simulink model "ZEPS"  (R2021b)
settings: Solver=VariableStepAuto  StartTime=0.0  StopTime=432000  FixedStep=1/60/60  RelTol=1e-3
model workspace: external: MATLAB File modelWorkspace.m (data not in the file)
values from neighbouring files (symbols this model uses):
  controlBT = 1    [modelWorkspace.m]
  controlEng = 1    [modelWorkspace.m]
  controlFC = 0    [modelWorkspace.m]
  controlFW = 0    [modelWorkspace.m]
  controlHS = 1    [modelWorkspace.m]
  controlSol = 0    [modelWorkspace.m]
  controlW = 0    [modelWorkspace.m]
  controlWW = 0    [modelWorkspace.m]
  data = get_scenario(scenario)    [UpdateModel.m]    (also in f_import_PEL.m = rmmissing(data,1,'MinNumMissing',10); get_scenario.m = data(timerange(datetime(FROM, 'InputFormat', 'dd.MM.yyyy HH:; thesis_images.m = get_scenario(1))
  sun = sun(sun.Date>date,:)    [get_irradiance.m]    (also in get_solar_from_file.m = sun(timerange(FROM+dt, TO+dt),:); thesis_images.m = get_irradiance(50, 14, "01.01.2016"))
undefined symbols (not defined in the file or in its folder): days, Ion, Lithium, seconds
libraries: mylib x15, simulink x5, spsControlledCurrentSourceLib x5, spsVoltageMeasurementLib x5, spsBatteryLib x1, simulink_extras x1, spspowerguiLib x1
settings Model: PacingRate=3600  VariantFading=off  Creator=janluca  LastModifiedBy=janluca
settings SolverCC: ZeroCrossAlgorithm=Adaptive  AlgebraicLoopSolver=LineSearch
settings DebuggingCC: AlgebraicLoopMsg=none  IgnoredZcDiagnostic=none  SFMachineParentedDataDiag=warning

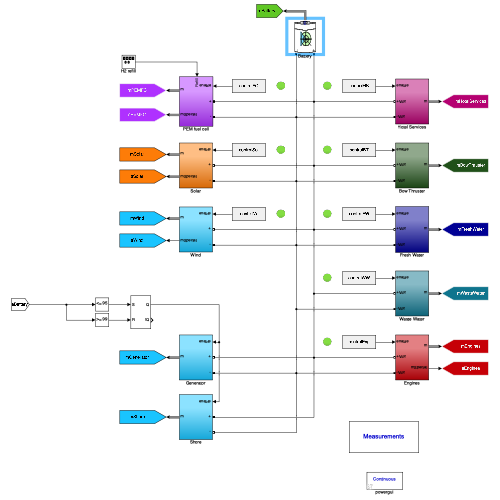
[thumbnail: Simulink's stored preview of the top-level diagram]
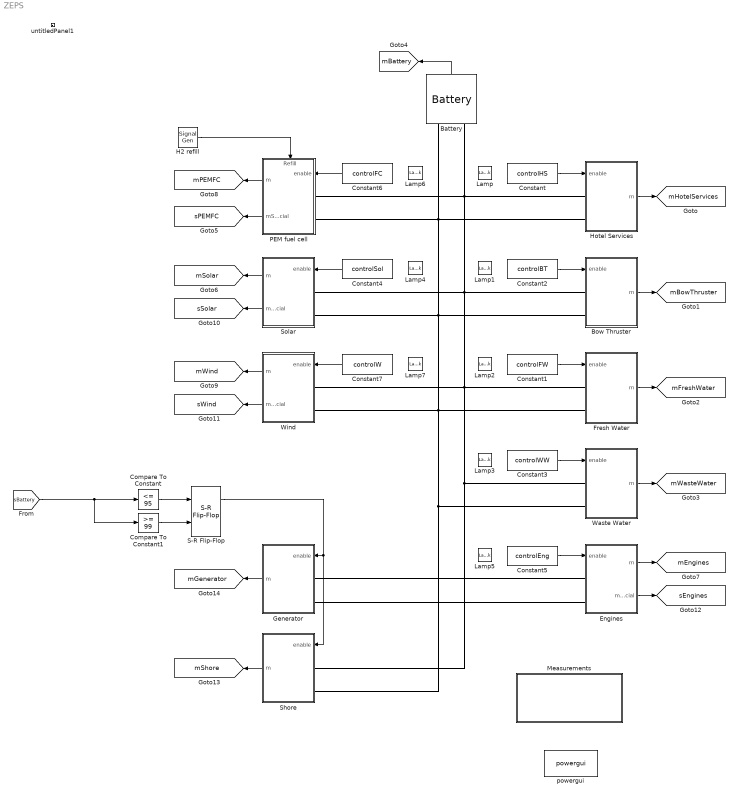
== system ZEPS ==
  Battery : spsBatteryLib/Battery  BatType=Lithium-Ion  ShowTempParam=off  ThermalPreset=no  ShowAgeParam=off  NomV=38.4*21  NomQ=100*50  SOC=90  Batt_Tr=0.1  PresetModel=off  MaxQ=125*50  MinV=30*21  FullV=42*21  Dis_rate=50*50  R=0.0024828  Normal_OP=100*50  expZone=[837.9 2500]  current=[20 100 200]  Units=Time  Tci=20  NomT=20  T2=-30  MaxQ2=4.8  FullV2=7.1  Normal_OP2=5.655  expZone2="[6.58           1]"  Rca=0.6  ti=2000  Dp=0  Neq0=0  Tsim=1e6  Ta1=25  Qeol=5.4*0.9  Reol=0.013333*1.2  Char_age=[2.3478, 3]  Dis_age=[2.3478, 10]  N1=1500  N2=10500  N3=1000  N4=1400  Ta2=45  N5=950
  Bow Thruster : Subsystem
  Compare To Constant : simulink/Logic and Bit Operations/Compare To Constant  relop=<=  const=95  OutDataTypeStr=boolean
  Compare To Constant1 : simulink/Logic and Bit Operations/Compare To Constant  relop=>=  const=99  OutDataTypeStr=boolean
  Constant : Constant  Value=controlHS
  Constant1 : Constant  Value=controlFW
  Constant2 : Constant  Value=controlBT
  Constant3 : Constant  Value=controlWW
  Constant4 : Constant  Value=controlSol
  Constant5 : Constant  Value=controlEng
  Constant6 : Constant  Value=controlFC
  Constant7 : Constant  Value=controlW
  Engines : Subsystem
  Fresh Water : Subsystem
  Generator : Subsystem
      settings: PortSchema="{\"entries\":[{\"content\":{\"sides\":[{\"content\":{\"connectorIds\":[\"Out1\"]},\"type\":\"ConnectorPlacement.EquallySpacedRectSide\",\"uuid\":\"11c6df83-a77d-42e1-93c3-7e92626e8295\"},{\"content\":{\"connectorIds\":[\"In1\",\"RConn1\",\"RConn2\"],\"side\":\"RIGHT\"},\"type\":\"ConnectorPlacement.EquallySpacedRectSide\",\"uuid\":\"be484aa3-b470-4b9a-a56f-17a6492ffa37\"},{\"content\":{\"connectorIds\":[],\"side\":\"TOP\"},\"type\":\"ConnectorPlacement.EquallySpacedRectSide\",\"uuid\":\"b9721f03-f883-4f0f-ae4c-83e5c2ad9b8b\"},{\"content\":{\"connectorIds\":[],\"side\":\"HIDDEN\"},\"type\":\"ConnectorPlacement.EquallySpacedRectSide\",\"uuid\":\"b91deee7-9db2-4cb3-a16e-378b8e6a58a6\"}]},\"type\":\"ConnectorPlacement.EquallySpacedConnector\",\"uuid\":\"590b808f-ca80-4a0b-b9c9-4d18c7197559\"}],\"packageUris\":[\"http://schema.mathworks.com/mf0/Connector/R2020b\"],\"version\":\"1.0\"}"
  H2 refill : SignalGenerator  WaveForm=sawtooth  Amplitude=0  Frequency=1/seconds(days(1))
  Hotel Services : Subsystem
  Lamp{,1..7} (8 alike) : LampBlock  LabelPosition=Hide
  Measurements : Subsystem
      mask Display: color('blue');disp('Measurements')
  PEM fuel cell : Subsystem
      settings: PortSchema="{\"entries\":[{\"content\":{\"sides\":[{\"content\":{\"connectorIds\":[\"Out1\",\"Out2\"]},\"type\":\"ConnectorPlacement.EquallySpacedRectSide\",\"uuid\":\"11c6df83-a77d-42e1-93c3-7e92626e8295\"},{\"content\":{\"connectorIds\":[\"In2\",\"RConn1\",\"RConn2\"],\"side\":\"RIGHT\"},\"type\":\"ConnectorPlacement.EquallySpacedRectSide\",\"uuid\":\"be484aa3-b470-4b9a-a56f-17a6492ffa37\"},{\"content\":{\"connectorIds\":[\"In1\"],\"side\":\"TOP\"},\"type\":\"ConnectorPlacement.EquallySpacedRectSide\",\"uuid\":\"b9721f03-f883-4f0f-ae4c-83e5c2ad9b8b\"},{\"content\":{\"connectorIds\":[],\"side\":\"HIDDEN\"},\"type\":\"ConnectorPlacement.EquallySpacedRectSide\",\"uuid\":\"b91deee7-9db2-4cb3-a16e-378b8e6a58a6\"}]},\"type\":\"ConnectorPlacement.EquallySpacedConnector\",\"uuid\":\"590b808f-ca80-4a0b-b9c9-4d18c7197559\"}],\"packageUris\":[\"http://schema.mathworks.com/mf0/Connector/R2020b\"],\"version\":\"1.0\"}"
  S-R Flip-Flop : simulink_extras/Flip Flops/S-R Flip-Flop  initial_condition=0
  Shore : Subsystem
      settings: PortSchema="{\"entries\":[{\"content\":{\"sides\":[{\"content\":{\"connectorIds\":[\"Out1\"]},\"type\":\"ConnectorPlacement.EquallySpacedRectSide\",\"uuid\":\"11c6df83-a77d-42e1-93c3-7e92626e8295\"},{\"content\":{\"connectorIds\":[\"In1\",\"RConn1\",\"RConn2\"],\"side\":\"RIGHT\"},\"type\":\"ConnectorPlacement.EquallySpacedRectSide\",\"uuid\":\"be484aa3-b470-4b9a-a56f-17a6492ffa37\"},{\"content\":{\"connectorIds\":[],\"side\":\"TOP\"},\"type\":\"ConnectorPlacement.EquallySpacedRectSide\",\"uuid\":\"b9721f03-f883-4f0f-ae4c-83e5c2ad9b8b\"},{\"content\":{\"connectorIds\":[],\"side\":\"HIDDEN\"},\"type\":\"ConnectorPlacement.EquallySpacedRectSide\",\"uuid\":\"b91deee7-9db2-4cb3-a16e-378b8e6a58a6\"}]},\"type\":\"ConnectorPlacement.EquallySpacedConnector\",\"uuid\":\"590b808f-ca80-4a0b-b9c9-4d18c7197559\"}],\"packageUris\":[\"http://schema.mathworks.com/mf0/Connector/R2020b\"],\"version\":\"1.0\"}"
  Solar : Subsystem
      settings: PortSchema="{\"entries\":[{\"content\":{\"sides\":[{\"content\":{\"connectorIds\":[\"Out1\",\"Out2\"]},\"type\":\"ConnectorPlacement.EquallySpacedRectSide\",\"uuid\":\"11c6df83-a77d-42e1-93c3-7e92626e8295\"},{\"content\":{\"connectorIds\":[\"In1\",\"RConn1\",\"RConn2\"],\"side\":\"RIGHT\"},\"type\":\"ConnectorPlacement.EquallySpacedRectSide\",\"uuid\":\"be484aa3-b470-4b9a-a56f-17a6492ffa37\"},{\"content\":{\"connectorIds\":[],\"side\":\"TOP\"},\"type\":\"ConnectorPlacement.EquallySpacedRectSide\",\"uuid\":\"b9721f03-f883-4f0f-ae4c-83e5c2ad9b8b\"},{\"content\":{\"connectorIds\":[],\"side\":\"HIDDEN\"},\"type\":\"ConnectorPlacement.EquallySpacedRectSide\",\"uuid\":\"b91deee7-9db2-4cb3-a16e-378b8e6a58a6\"}]},\"type\":\"ConnectorPlacement.EquallySpacedConnector\",\"uuid\":\"590b808f-ca80-4a0b-b9c9-4d18c7197559\"}],\"packageUris\":[\"http://schema.mathworks.com/mf0/Connector/R2020b\"],\"version\":\"1.0\"}"
  Waste Water : Subsystem
  Wind : Subsystem
      settings: PortSchema="{\"entries\":[{\"content\":{\"sides\":[{\"content\":{\"connectorIds\":[\"Out1\",\"Out2\"]},\"type\":\"ConnectorPlacement.EquallySpacedRectSide\",\"uuid\":\"11c6df83-a77d-42e1-93c3-7e92626e8295\"},{\"content\":{\"connectorIds\":[\"In1\",\"RConn1\",\"RConn2\"],\"side\":\"RIGHT\"},\"type\":\"ConnectorPlacement.EquallySpacedRectSide\",\"uuid\":\"be484aa3-b470-4b9a-a56f-17a6492ffa37\"},{\"content\":{\"connectorIds\":[],\"side\":\"TOP\"},\"type\":\"ConnectorPlacement.EquallySpacedRectSide\",\"uuid\":\"b9721f03-f883-4f0f-ae4c-83e5c2ad9b8b\"},{\"content\":{\"connectorIds\":[],\"side\":\"HIDDEN\"},\"type\":\"ConnectorPlacement.EquallySpacedRectSide\",\"uuid\":\"b91deee7-9db2-4cb3-a16e-378b8e6a58a6\"}]},\"type\":\"ConnectorPlacement.EquallySpacedConnector\",\"uuid\":\"590b808f-ca80-4a0b-b9c9-4d18c7197559\"}],\"packageUris\":[\"http://schema.mathworks.com/mf0/Connector/R2020b\"],\"version\":\"1.0\"}"
  powergui : spspowerguiLib/powergui  Priority=1  SimulationMode=Continuous  SampleTime=60  frequency=60  Iterations=50  frequencyindice=0  Pbase=100e6  ErrMax=1e-4  UnitsV=kV  UnitsW=MW  buscounter=0  FunctionMessages=off  echomessages=off  EnableUseOfTLC=off  CurrentSourceSwitches=off  DisableSnubberDevices=off  DisableRonSwitches=off  DisableVfSwitches=off  DisplayEquations=off  AutomaticDiscreteSolvers=off  SolverType=Tustin/Backward Euler (TBE)  Interpol=off  ExternalGateDelay=off  methode=off  Ts=100  x0status=blocks  SPID=on  SwTol=0  HookPort=off  NonlinearTolerance=1e-4  nMaxIteration=100  ContinueOnMaxIteration=off  RestoreLinks=warning  ResistiveCurrentMeasurement=off  Frange=[0:2:500]  Ylog=off  Xlog=on  ShowGrid=off  save=off  variable=ZData  structure=0  ZoomFFT=off  StartTime=0.0  cycles=1  DisplayStyle=1  fundamental=60  FreqAxis=off  MaxFrequency=1000  frequencyindicesteady=1  RmsSteady=1  display=off
  untitledPanel1 : Subsystem  Tag=HiddenForWebPanel  IsWebBlockPanel=on
  tag scope: mBattery=global, mBowThruster=global, mEngines=global, mFreshWater=global, mGenerator=global, mHotelServices=global, mPEMFC=global, mShore=global, mSolar=global, mWasteWater=global, mWind=global, sEngines=global, sPEMFC=global, sSolar=global, sWind=global
  wires:
  Constant/1 -> Hotel Services/1(enable)
  Hotel Services/1(m) -> [mHotelServices]
  Bow Thruster/1(m) -> [mBowThruster]
  Fresh Water/1(m) -> [mFreshWater]
  Waste Water/1(m) -> [mWasteWater]
  Battery/1 -> [mBattery]
  Constant2/1 -> Bow Thruster/1(enable)
  Constant1/1 -> Fresh Water/1(enable)
  Constant3/1 -> Waste Water/1(enable)
  Solar/1(m) -> [mSolar]
  Constant4/1 -> Solar/1(enable)
  Constant5/1 -> Engines/1(enable)
  Engines/1(m) -> [mEngines]
  PEM fuel cell/1(m) -> [mPEMFC]
  Constant6/1 -> PEM fuel cell/2(enable)
  Wind/1(m) -> [mWind]
  Constant7/1 -> Wind/1(enable)
  PEM fuel cell/2(mSpecial) -> [sPEMFC]
  Solar/2(mSpecial) -> [sSolar]
  Wind/2(mSpecial) -> [sWind]
  Engines/2(mSpecial) -> [sEngines]
  H2 refill/1 -> PEM fuel cell/1(Refill)
  Generator/1(m) -> [mGenerator]
  Compare To Constant/1 -> S-R Flip-Flop/1
  [sBattery] -> Compare To Constant1/1, Compare To Constant/1
  Compare To Constant1/1 -> S-R Flip-Flop/2
  S-R Flip-Flop/1 -> Shore/1(enable), Generator/1(enable)
  Shore/1(m) -> [mShore]
  connections:
  Hotel Services/LConn1 -- Shore/RConn1 -- Engines/LConn1 -- Generator/RConn1 -- Waste Water/LConn1 -- Wind/RConn1 -- Fresh Water/LConn1 -- Solar/RConn1 -- Bow Thruster/LConn1 -- PEM fuel cell/RConn1 -- Battery/LConn1
  Hotel Services/LConn2 -- Wind/RConn2 -- Shore/RConn2 -- Engines/LConn2 -- Generator/RConn2 -- Waste Water/LConn2 -- Fresh Water/LConn2 -- Solar/RConn2 -- Bow Thruster/LConn2 -- PEM fuel cell/RConn2 -- Battery/LConn2

== system ZEPS/Bow Thruster ==
  enable : Inport
  AC converter simple : mylib/AC converter simple  eff=0.98
  Clock : Clock
  Constant : Constant  Value=0
  Load Data power bow thruster : Lookup_n-D  NumberOfTableDimensions=1  BreakpointsForDimension1=data.time  BeginIndexSearchUsingPreviousIndexResult=on  Table=data.P_BT  InternalRulePriority=Speed  RndMeth=Simplest  InputSameDT=on
  Switch : Switch  Criteria=u2 > Threshold
  VI measurement : mylib/VI measurement  SystemSampleTime=-1  VariantActivationTime=update diagram  Latency=0  AutoFrameSizeCalculation=off
      settings: PortSchema="{\"entries\":[{\"content\":{\"sides\":[{\"content\":{\"connectorIds\":[\"LConn1\",\"LConn2\"]},\"type\":\"ConnectorPlacement.EquallySpacedRectSide\",\"uuid\":\"f3b73344-d0cf-4b93-ad96-f780fa5a1256\"},{\"content\":{\"connectorIds\":[\"RConn1\",\"RConn2\"],\"side\":\"RIGHT\"},\"type\":\"ConnectorPlacement.EquallySpacedRectSide\",\"uuid\":\"030ebb8c-daa3-4185-a78c-b002204e2a62\"},{\"content\":{\"connectorIds\":[\"Out1\"],\"side\":\"TOP\"},\"type\":\"ConnectorPlacement.EquallySpacedRectSide\",\"uuid\":\"0cc05069-4c24-40a7-976e-8b87ed915541\"},{\"content\":{\"connectorIds\":[],\"side\":\"HIDDEN\"},\"type\":\"ConnectorPlacement.EquallySpacedRectSide\",\"uuid\":\"da030f82-010e-483f-97d7-c36c3edfce40\"}]},\"type\":\"ConnectorPlacement.EquallySpacedConnector\",\"uuid\":\"1bb0f634-fa5d-4f47-8259-a0e02a201bbc\"}],\"packageUris\":[\"http://schema.mathworks.com/mf0/Connector/R2020b\"],\"version\":\"1.0\"}"
  +Vdc : PMIOPort  Tag=PMCPort  Side=Left
  -Vdc : PMIOPort  Tag=PMCPort  Port=2  Side=Left
  m : Outport
  wires:
  Switch/1 -> AC converter simple/1
  VI measurement/1 -> m/1
  Clock/1 -> Load Data power bow thruster/1
  enable/1 -> Switch/2
  Constant/1 -> Switch/3
  Load Data power bow thruster/1 -> Switch/1
  connections:
  VI measurement/LConn1 -- AC converter simple/RConn1
  +Vdc/RConn1 -- VI measurement/RConn1
  -Vdc/RConn1 -- VI measurement/RConn2
  VI measurement/LConn2 -- AC converter simple/RConn2

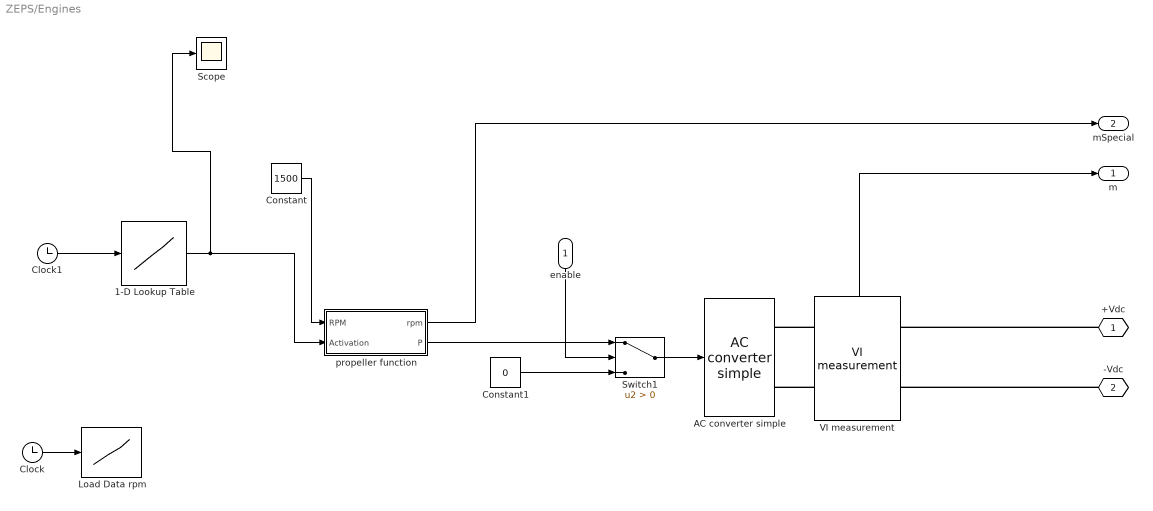
== system ZEPS/Engines ==
  enable : Inport
  1-D Lookup Table : Lookup_n-D  NumberOfTableDimensions=1  BreakpointsForDimension1="3600* [0   2    21    24    43    49    68    72    91    97   116   119   138   143]"  Table="600*[1    0    1     0     1     0     1     0     1     0     1     0     1     0]"  InterpMethod=Flat  InternalRulePriority=Speed  RndMeth=Simplest  InputSameDT=on
  AC converter simple : mylib/AC converter simple  eff=0.98
  Clock : Clock
  Clock1 : Clock
  Constant : Constant  Value=1500
  Constant1 : Constant  Value=0
  Load Data rpm : Lookup_n-D  NumberOfTableDimensions=1  BreakpointsForDimension1=data.time  BeginIndexSearchUsingPreviousIndexResult=on  Table=data.rpm  InternalRulePriority=Speed  RndMeth=Simplest  InputSameDT=on
  Scope : Scope
  Switch1 : Switch  Criteria=u2 > Threshold
  VI measurement : mylib/VI measurement  SystemSampleTime=-1  VariantActivationTime=update diagram  Latency=0  AutoFrameSizeCalculation=off
      settings: PortSchema="{\"entries\":[{\"content\":{\"sides\":[{\"content\":{\"connectorIds\":[\"LConn1\",\"LConn2\"]},\"type\":\"ConnectorPlacement.EquallySpacedRectSide\",\"uuid\":\"f3b73344-d0cf-4b93-ad96-f780fa5a1256\"},{\"content\":{\"connectorIds\":[\"RConn1\",\"RConn2\"],\"side\":\"RIGHT\"},\"type\":\"ConnectorPlacement.EquallySpacedRectSide\",\"uuid\":\"030ebb8c-daa3-4185-a78c-b002204e2a62\"},{\"content\":{\"connectorIds\":[\"Out1\"],\"side\":\"TOP\"},\"type\":\"ConnectorPlacement.EquallySpacedRectSide\",\"uuid\":\"0cc05069-4c24-40a7-976e-8b87ed915541\"},{\"content\":{\"connectorIds\":[],\"side\":\"HIDDEN\"},\"type\":\"ConnectorPlacement.EquallySpacedRectSide\",\"uuid\":\"da030f82-010e-483f-97d7-c36c3edfce40\"}]},\"type\":\"ConnectorPlacement.EquallySpacedConnector\",\"uuid\":\"1bb0f634-fa5d-4f47-8259-a0e02a201bbc\"}],\"packageUris\":[\"http://schema.mathworks.com/mf0/Connector/R2020b\"],\"version\":\"1.0\"}"
  propeller function : Subsystem
  +Vdc : PMIOPort  Tag=PMCPort  Side=Left
  -Vdc : PMIOPort  Tag=PMCPort  Port=2  Side=Left
  m : Outport
  mSpecial : Outport  Port=2
  wires:
  Clock/1 -> Load Data rpm/1
  Switch1/1 -> AC converter simple/1
  Constant1/1 -> Switch1/3
  propeller function/2(P) -> Switch1/1
  enable/1 -> Switch1/2
  VI measurement/1 -> m/1
  propeller function/1(rpm) -> mSpecial/1
  Clock1/1 -> 1-D Lookup Table/1
  Constant/1 -> propeller function/1(RPM)
  1-D Lookup Table/1 -> propeller function/2(Activation), Scope/1
  connections:
  VI measurement/LConn1 -- AC converter simple/RConn1
  -Vdc/RConn1 -- VI measurement/RConn2
  VI measurement/LConn2 -- AC converter simple/RConn2
  +Vdc/RConn1 -- VI measurement/RConn1

== system ZEPS/Fresh Water ==
  enable : Inport
  AC converter simple : mylib/AC converter simple  eff=0.98
  Constant : Constant  Value=0
  Power : Constant  Value=2300
  Switch : Switch  Criteria=u2 > Threshold
  VI measurement : mylib/VI measurement  SystemSampleTime=-1  VariantActivationTime=update diagram  Latency=0  AutoFrameSizeCalculation=off
      settings: PortSchema="{\"entries\":[{\"content\":{\"sides\":[{\"content\":{\"connectorIds\":[\"LConn1\",\"LConn2\"]},\"type\":\"ConnectorPlacement.EquallySpacedRectSide\",\"uuid\":\"f3b73344-d0cf-4b93-ad96-f780fa5a1256\"},{\"content\":{\"connectorIds\":[\"RConn1\",\"RConn2\"],\"side\":\"RIGHT\"},\"type\":\"ConnectorPlacement.EquallySpacedRectSide\",\"uuid\":\"030ebb8c-daa3-4185-a78c-b002204e2a62\"},{\"content\":{\"connectorIds\":[\"Out1\"],\"side\":\"TOP\"},\"type\":\"ConnectorPlacement.EquallySpacedRectSide\",\"uuid\":\"0cc05069-4c24-40a7-976e-8b87ed915541\"},{\"content\":{\"connectorIds\":[],\"side\":\"HIDDEN\"},\"type\":\"ConnectorPlacement.EquallySpacedRectSide\",\"uuid\":\"da030f82-010e-483f-97d7-c36c3edfce40\"}]},\"type\":\"ConnectorPlacement.EquallySpacedConnector\",\"uuid\":\"1bb0f634-fa5d-4f47-8259-a0e02a201bbc\"}],\"packageUris\":[\"http://schema.mathworks.com/mf0/Connector/R2020b\"],\"version\":\"1.0\"}"
  +Vdc : PMIOPort  Tag=PMCPort  Side=Left
  -Vdc : PMIOPort  Tag=PMCPort  Port=2  Side=Left
  m : Outport
  wires:
  VI measurement/1 -> m/1
  enable/1 -> Switch/2
  Constant/1 -> Switch/3
  Power/1 -> Switch/1
  Switch/1 -> AC converter simple/1
  connections:
  VI measurement/LConn1 -- AC converter simple/RConn1
  VI measurement/LConn2 -- AC converter simple/RConn2
  +Vdc/RConn1 -- VI measurement/RConn1
  -Vdc/RConn1 -- VI measurement/RConn2

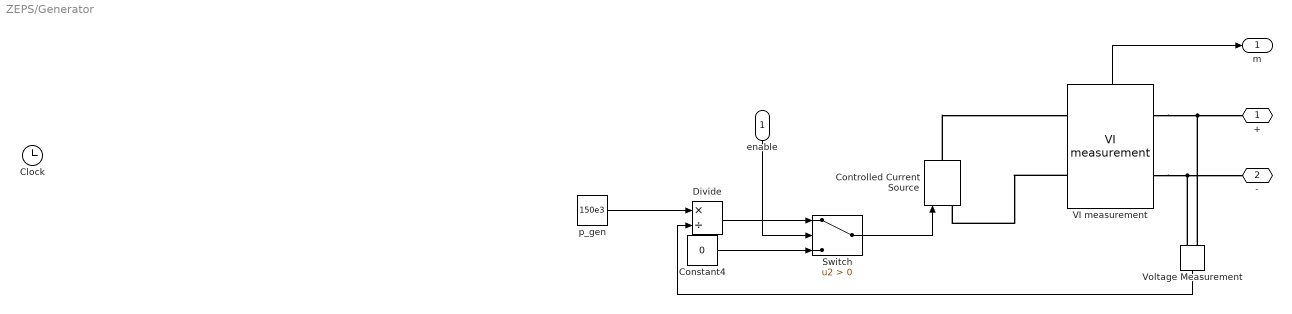
== system ZEPS/Generator ==
  enable : Inport
  Clock : Clock
  Constant4 : Constant  Value=0
  Controlled Current Source : spsControlledCurrentSourceLib/Controlled Current Source  Initialize=on  Source_Type=AC  Amplitude=0  Phase=0  Frequency=0  Measurements=None
  Divide : Product  Inputs=*/
  Switch : Switch  Criteria=u2 > Threshold
  VI measurement : mylib/VI measurement  SystemSampleTime=-1  VariantActivationTime=update diagram  Latency=0  AutoFrameSizeCalculation=off
      settings: PortSchema="{\"entries\":[{\"content\":{\"sides\":[{\"content\":{\"connectorIds\":[\"LConn1\",\"LConn2\"]},\"type\":\"ConnectorPlacement.EquallySpacedRectSide\",\"uuid\":\"f3b73344-d0cf-4b93-ad96-f780fa5a1256\"},{\"content\":{\"connectorIds\":[\"RConn1\",\"RConn2\"],\"side\":\"RIGHT\"},\"type\":\"ConnectorPlacement.EquallySpacedRectSide\",\"uuid\":\"030ebb8c-daa3-4185-a78c-b002204e2a62\"},{\"content\":{\"connectorIds\":[\"Out1\"],\"side\":\"TOP\"},\"type\":\"ConnectorPlacement.EquallySpacedRectSide\",\"uuid\":\"0cc05069-4c24-40a7-976e-8b87ed915541\"},{\"content\":{\"connectorIds\":[],\"side\":\"HIDDEN\"},\"type\":\"ConnectorPlacement.EquallySpacedRectSide\",\"uuid\":\"da030f82-010e-483f-97d7-c36c3edfce40\"}]},\"type\":\"ConnectorPlacement.EquallySpacedConnector\",\"uuid\":\"1bb0f634-fa5d-4f47-8259-a0e02a201bbc\"}],\"packageUris\":[\"http://schema.mathworks.com/mf0/Connector/R2020b\"],\"version\":\"1.0\"}"
  Voltage Measurement : spsVoltageMeasurementLib/Voltage Measurement  PhasorSimulation=off  OutputType=Complex  PSBequivalent=0
  p_gen : Constant  Value=150e3
  + : PMIOPort  Side=Right
  - : PMIOPort  Port=2  Side=Right
  m : Outport
  wires:
  Switch/1 -> Controlled Current Source/1
  enable/1 -> Switch/2
  Constant4/1 -> Switch/3
  Divide/1 -> Switch/1
  VI measurement/1 -> m/1
  Voltage Measurement/1 -> Divide/2
  p_gen/1 -> Divide/1
  connections:
  VI measurement/LConn1 -- Voltage Measurement/LConn1 -- +/RConn1
  VI measurement/LConn2 -- Voltage Measurement/LConn2 -- -/RConn1
  VI measurement/RConn2 -- Controlled Current Source/LConn1
  Controlled Current Source/RConn1 -- VI measurement/RConn1

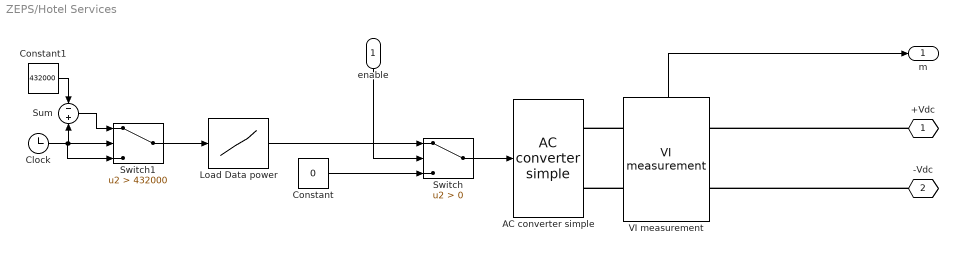
== system ZEPS/Hotel Services ==
  enable : Inport
  AC converter simple : mylib/AC converter simple  eff=0.98
  Clock : Clock
  Constant : Constant  Value=0
  Constant1 : Constant  Value=432000
  Load Data power : Lookup_n-D  NumberOfTableDimensions=1  BreakpointsForDimension1=data.time  BeginIndexSearchUsingPreviousIndexResult=on  Table=data.P  InternalRulePriority=Speed  RndMeth=Simplest  InputSameDT=on
  Sum : Sum  Inputs=-|+
  Switch : Switch  Criteria=u2 > Threshold
  Switch1 : Switch  Criteria=u2 > Threshold  Threshold=432000
  VI measurement : mylib/VI measurement  SystemSampleTime=-1  VariantActivationTime=update diagram  Latency=0  AutoFrameSizeCalculation=off
      settings: PortSchema="{\"entries\":[{\"content\":{\"sides\":[{\"content\":{\"connectorIds\":[\"LConn1\",\"LConn2\"]},\"type\":\"ConnectorPlacement.EquallySpacedRectSide\",\"uuid\":\"f3b73344-d0cf-4b93-ad96-f780fa5a1256\"},{\"content\":{\"connectorIds\":[\"RConn1\",\"RConn2\"],\"side\":\"RIGHT\"},\"type\":\"ConnectorPlacement.EquallySpacedRectSide\",\"uuid\":\"030ebb8c-daa3-4185-a78c-b002204e2a62\"},{\"content\":{\"connectorIds\":[\"Out1\"],\"side\":\"TOP\"},\"type\":\"ConnectorPlacement.EquallySpacedRectSide\",\"uuid\":\"0cc05069-4c24-40a7-976e-8b87ed915541\"},{\"content\":{\"connectorIds\":[],\"side\":\"HIDDEN\"},\"type\":\"ConnectorPlacement.EquallySpacedRectSide\",\"uuid\":\"da030f82-010e-483f-97d7-c36c3edfce40\"}]},\"type\":\"ConnectorPlacement.EquallySpacedConnector\",\"uuid\":\"1bb0f634-fa5d-4f47-8259-a0e02a201bbc\"}],\"packageUris\":[\"http://schema.mathworks.com/mf0/Connector/R2020b\"],\"version\":\"1.0\"}"
  +Vdc : PMIOPort  Tag=PMCPort  Side=Left
  -Vdc : PMIOPort  Tag=PMCPort  Port=2  Side=Left
  m : Outport
  wires:
  Load Data power/1 -> Switch/1
  enable/1 -> Switch/2
  Switch/1 -> AC converter simple/1
  VI measurement/1 -> m/1
  Constant/1 -> Switch/3
  Clock/1 -> Sum/2, Switch1/2, Switch1/3
  Switch1/1 -> Load Data power/1
  Sum/1 -> Switch1/1
  Constant1/1 -> Sum/1
  connections:
  VI measurement/LConn1 -- AC converter simple/RConn1
  VI measurement/LConn2 -- AC converter simple/RConn2
  +Vdc/RConn1 -- VI measurement/RConn1
  -Vdc/RConn1 -- VI measurement/RConn2

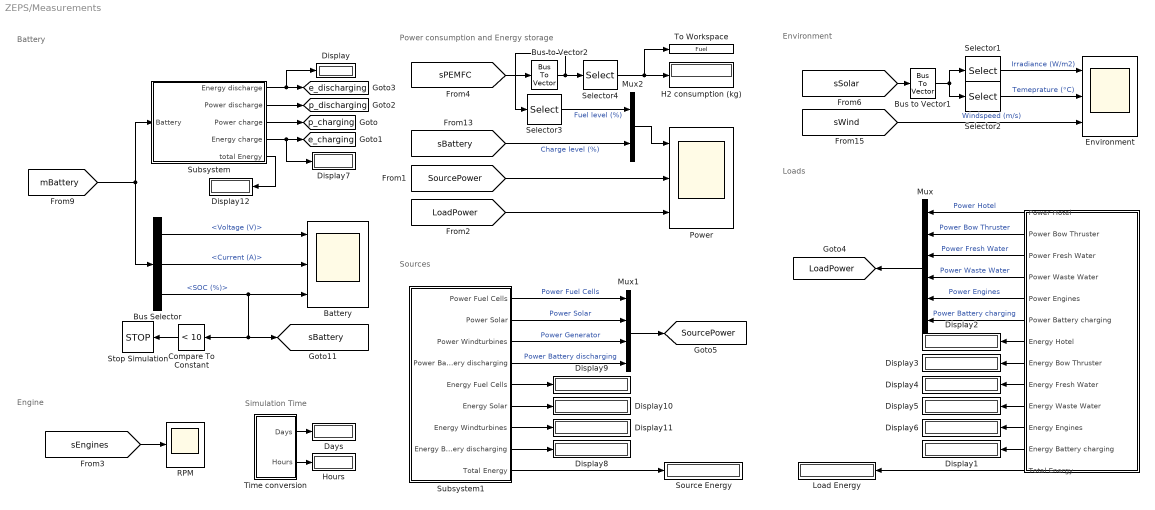
== system ZEPS/Measurements ==
  note: Engine
  note: Environment
  note: Power consumption and Energy storage
  note: Sources
  note: Loads
  note: Simulation Time
  note: Battery
  " " : Subsystem
  Battery : Scope  NumInputPorts=3
  Bus Selector : BusSelector  OutputSignals=Voltage (V),Current (A),SOC (%)
  Bus to Vector1 : BusToVector
  Bus to Vector2 : BusToVector
  Compare To Constant : simulink/Logic and Bit Operations/Compare To Constant  relop=<  const=10  OutDataTypeStr=boolean
  Days : Display
      settings: Format=bank
  Display{,1..12} (13 alike) : Display
  Environment : Scope  NumInputPorts=3
  H2 consumption (kg) : Display
  Hours : Display
      settings: Format=bank
  Load Energy : Display
      settings: Format=bank
  Mux : Mux  Inputs=6
  Mux1 : Mux
  Mux2 : Mux  Inputs=2
  Power : Scope  NumInputPorts=3
  RPM : Scope
  Selector1 : Selector  InputPortWidth=2  IndexOptions=Index vector (dialog)  Indices=1  OutputSizes=1
  Selector2 : Selector  InputPortWidth=2  IndexOptions=Index vector (dialog)  Indices=2  OutputSizes=1
  Selector3 : Selector  InputPortWidth=2  IndexOptions=Index vector (dialog)  Indices=2  OutputSizes=1
  Selector4 : Selector  InputPortWidth=2  IndexOptions=Index vector (dialog)  Indices=1  OutputSizes=1
  Source Energy : Display
      settings: Format=bank
  Stop Simulation : Stop
  Subsystem : Subsystem
  Subsystem1 : Subsystem
  Time conversion : Subsystem
  To Workspace : ToWorkspace  VariableName=Fuel  SaveFormat=Timeseries  SampleTime=-1
      settings: MaxDataPoints=1
  tag scope: LoadPower=global, SourcePower=global, e_charging=global, e_discharging=global, p_charging=global, p_discharging=global, sBattery=global
  wires:
  [mBattery] -> Subsystem/1(Battery), Bus Selector/1
  Bus Selector/3 -> Compare To Constant/1, [sBattery], Battery/3  "<SOC (%)>"
  Bus Selector/2 -> Battery/2  "<Current (A)>"
  Bus Selector/1 -> Battery/1  "<Voltage (V)>"
  Compare To Constant/1 -> Stop Simulation/1
  Subsystem/1(Energy discharge) -> [e_discharging], Display/1
  Subsystem/4(Energy charge) -> [e_charging], Display7/1
  Subsystem/3(Power charge) -> [p_charging]
  Subsystem/2(Power discharge) -> [p_discharging]
  Subsystem/5(total Energy) -> Display12/1
  Mux2/1 -> Power/1
  Selector2/1 -> Environment/2  "Temeprature (°C)"
  [sSolar] -> Bus to Vector1/1
  [sPEMFC] -> Bus to Vector2/1
  [sEngines] -> RPM/1
  Selector1/1 -> Environment/1  "Irradiance (W/m2)"
  [sWind] -> Environment/3  "Windspeed (m/s)"
  [sBattery] -> Mux2/2  "Charge level (%)"
  Selector3/1 -> Mux2/1  "Fuel level (%)"
  Bus to Vector1/1 -> Selector2/1, Selector1/1
  " "/1(Power Hotel) -> Mux/1  "Power Hotel"
  " "/2(Power Bow Thruster) -> Mux/2  "Power Bow Thruster"
  " "/3(Power Fresh Water) -> Mux/3  "Power Fresh Water"
  " "/4(Power Waste Water) -> Mux/4  "Power Waste Water"
  " "/5(Power Engines) -> Mux/5  "Power Engines"
  " "/7(Energy Hotel) -> Display2/1
  " "/8(Energy Bow Thruster) -> Display3/1
  " "/9(Energy Fresh Water) -> Display4/1
  " "/10(Energy Waste Water) -> Display5/1
  " "/11(Energy Engines) -> Display6/1
  " "/6(Power Battery charging) -> Mux/6  "Power Battery charging"
  " "/12(Energy Battery charging) -> Display1/1
  " "/13(Total Energy) -> Load Energy/1
  Mux/1 -> [LoadPower]
  Subsystem1/1(Power Fuel Cells) -> Mux1/1  "Power Fuel Cells"
  Subsystem1/2(Power Solar) -> Mux1/2  "Power Solar"
  Subsystem1/3(Power Windturbines) -> Mux1/3  "Power Generator"
  Subsystem1/4(Power Battery discharging) -> Mux1/4  "Power Battery discharging"
  Subsystem1/5(Energy Fuel Cells) -> Display9/1
  Subsystem1/6(Energy Solar) -> Display10/1
  Subsystem1/7(Energy Windturbines) -> Display11/1
  Subsystem1/8(Energy Battery discharging) -> Display8/1
  Subsystem1/9(Total Energy) -> Source Energy/1
  Mux1/1 -> [SourcePower]
  [SourcePower] -> Power/2
  [LoadPower] -> Power/3
  Selector4/1 -> To Workspace/1, H2 consumption (kg)/1
  Time conversion/1(Days) -> Days/1
  Time conversion/2(Hours) -> Hours/1
  Bus to Vector2/1 -> Selector3/1, Selector4/1

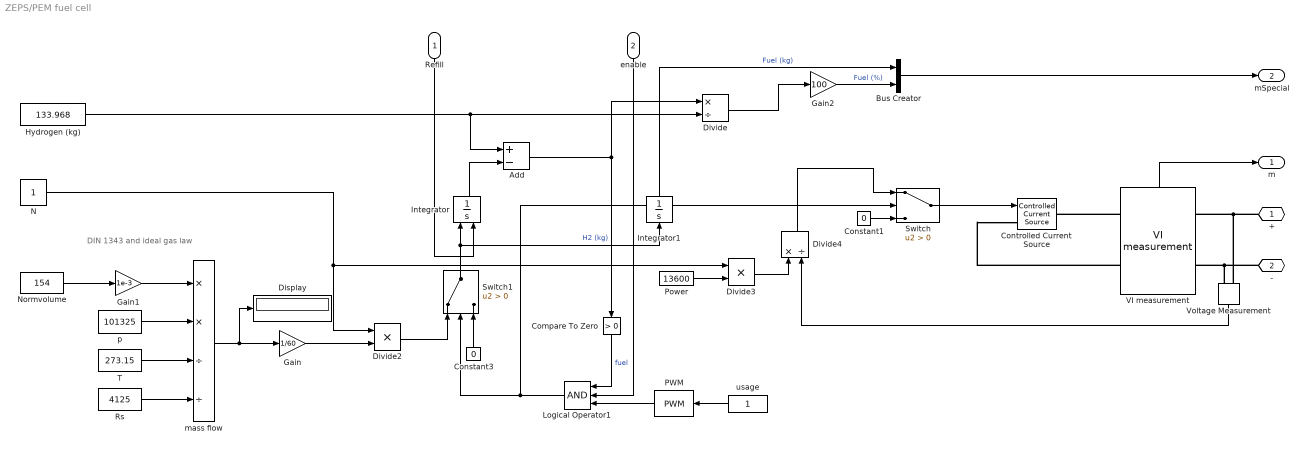
== system ZEPS/PEM fuel cell ==
  note: DIN 1343 and ideal gas law
  Refill : Inport
  enable : Inport  Port=2
  Add : Sum  Inputs=+-
  Bus Creator : BusCreator  Inputs=2
  Compare To Zero : simulink/Logic and Bit Operations/Compare To Zero  relop=>  OutDataTypeStr=boolean
  Constant1 : Constant  Value=0
  Constant3 : Constant  Value=0
  Controlled Current Source : spsControlledCurrentSourceLib/Controlled Current Source  Initialize=on  Source_Type=AC  Amplitude=0  Phase=0  Frequency=0  Measurements=None
  Display : Display
  Divide : Product  Inputs=*/
  Divide2 : Product  Inputs=**
  Divide3 : Product  Inputs=**
  Divide4 : Product  Inputs=*/
  Gain : Gain  Gain=1/60
  Gain1 : Gain  Gain=1e-3
  Gain2 : Gain  Gain=100
  Hydrogen (kg) : Constant  Value=133.968
  Integrator : Integrator  ExternalReset=rising
  Integrator1 : Integrator
  Logical Operator1 : Logic  Inputs=3  AllPortsSameDT=off  OutDataTypeStr=boolean
  N : Constant
  Normvolume : Constant  Value=154
  PWM : simulink/Discontinuities/PWM  DisableCoverage=on  Period=12*3600  DisallowZeroDutyCycle=off  RunAtFixedTimeIntervals=off  SampleTime=0.1
  Power : Constant  Value=13600
  Rs : Constant  Value=4125
  Switch : Switch  Criteria=u2 > Threshold
  Switch1 : Switch  Criteria=u2 > Threshold
  T : Constant  Value=273.15
  VI measurement : mylib/VI measurement  SystemSampleTime=-1  VariantActivationTime=update diagram  Latency=0  AutoFrameSizeCalculation=off
      settings: PortSchema="{\"entries\":[{\"content\":{\"sides\":[{\"content\":{\"connectorIds\":[\"LConn1\",\"LConn2\"]},\"type\":\"ConnectorPlacement.EquallySpacedRectSide\",\"uuid\":\"f3b73344-d0cf-4b93-ad96-f780fa5a1256\"},{\"content\":{\"connectorIds\":[\"RConn1\",\"RConn2\"],\"side\":\"RIGHT\"},\"type\":\"ConnectorPlacement.EquallySpacedRectSide\",\"uuid\":\"030ebb8c-daa3-4185-a78c-b002204e2a62\"},{\"content\":{\"connectorIds\":[\"Out1\"],\"side\":\"TOP\"},\"type\":\"ConnectorPlacement.EquallySpacedRectSide\",\"uuid\":\"0cc05069-4c24-40a7-976e-8b87ed915541\"},{\"content\":{\"connectorIds\":[],\"side\":\"HIDDEN\"},\"type\":\"ConnectorPlacement.EquallySpacedRectSide\",\"uuid\":\"da030f82-010e-483f-97d7-c36c3edfce40\"}]},\"type\":\"ConnectorPlacement.EquallySpacedConnector\",\"uuid\":\"1bb0f634-fa5d-4f47-8259-a0e02a201bbc\"}],\"packageUris\":[\"http://schema.mathworks.com/mf0/Connector/R2020b\"],\"version\":\"1.0\"}"
  Voltage Measurement : spsVoltageMeasurementLib/Voltage Measurement  PhasorSimulation=off  OutputType=Complex  PSBequivalent=0
  mass flow : Product  Inputs=**//
  p : Constant  Value=101325
  usage : Constant
  + : PMIOPort  Side=Right
  - : PMIOPort  Port=2  Side=Right
  m : Outport
  mSpecial : Outport  Port=2
  wires:
  Constant1/1 -> Switch/3
  Hydrogen (kg)/1 -> Add/1, Divide/2
  Add/1 -> Divide/1, Compare To Zero/1  "H2 (kg)"
  Constant3/1 -> Switch1/3
  Integrator/1 -> Add/2
  usage/1 -> PWM/1
  Switch1/1 -> Integrator/1, Integrator1/1
  VI measurement/1 -> m/1
  Switch/1 -> Controlled Current Source/1
  Divide2/1 -> Switch1/1
  Divide4/1 -> Switch/1
  Power/1 -> Divide3/2
  Voltage Measurement/1 -> Divide4/2
  Logical Operator1/1 -> Switch/2, Switch1/2
  Divide3/1 -> Divide4/1
  N/1 -> Divide2/1, Divide3/1
  mass flow/1 -> Display/1, Gain/1
  Refill/1 -> Integrator/2
  p/1 -> mass flow/2
  Normvolume/1 -> Gain1/1
  T/1 -> mass flow/3
  Rs/1 -> mass flow/4
  Gain/1 -> Divide2/2
  Divide/1 -> Gain2/1
  Bus Creator/1 -> mSpecial/1
  Gain1/1 -> mass flow/1
  Compare To Zero/1 -> Logical Operator1/1  "fuel"
  Gain2/1 -> Bus Creator/2  "Fuel (%)"
  enable/1 -> Logical Operator1/2
  Integrator1/1 -> Bus Creator/1  "Fuel (kg)"
  PWM/1 -> Logical Operator1/3
  connections:
  +/RConn1 -- Voltage Measurement/LConn1 -- VI measurement/LConn1
  -/RConn1 -- Voltage Measurement/LConn2 -- VI measurement/LConn2
  VI measurement/RConn1 -- Controlled Current Source/RConn1
  VI measurement/RConn2 -- Controlled Current Source/LConn1

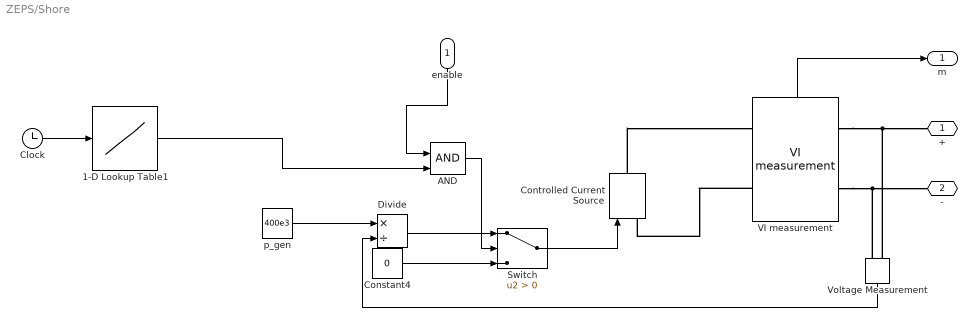
== system ZEPS/Shore ==
  enable : Inport
  1-D Lookup Table1 : Lookup_n-D  NumberOfTableDimensions=1  BreakpointsForDimension1="3600* [0   2    21    24    43    49    68    72    91    97   116   119   138   143]"  Table="[0     1   0    1     0     0     0     0    0     1     0     1     0     1]"  InterpMethod=Flat  InternalRulePriority=Speed  RndMeth=Simplest  InputSameDT=on
  AND : Logic  IconShape=distinctive  AllPortsSameDT=off  OutDataTypeStr=boolean
  Clock : Clock
  Constant4 : Constant  Value=0
  Controlled Current Source : spsControlledCurrentSourceLib/Controlled Current Source  Initialize=on  Source_Type=AC  Amplitude=0  Phase=0  Frequency=0  Measurements=None
  Divide : Product  Inputs=*/
  Switch : Switch  Criteria=u2 > Threshold
  VI measurement : mylib/VI measurement  SystemSampleTime=-1  VariantActivationTime=update diagram  Latency=0  AutoFrameSizeCalculation=off
      settings: PortSchema="{\"entries\":[{\"content\":{\"sides\":[{\"content\":{\"connectorIds\":[\"LConn1\",\"LConn2\"]},\"type\":\"ConnectorPlacement.EquallySpacedRectSide\",\"uuid\":\"f3b73344-d0cf-4b93-ad96-f780fa5a1256\"},{\"content\":{\"connectorIds\":[\"RConn1\",\"RConn2\"],\"side\":\"RIGHT\"},\"type\":\"ConnectorPlacement.EquallySpacedRectSide\",\"uuid\":\"030ebb8c-daa3-4185-a78c-b002204e2a62\"},{\"content\":{\"connectorIds\":[\"Out1\"],\"side\":\"TOP\"},\"type\":\"ConnectorPlacement.EquallySpacedRectSide\",\"uuid\":\"0cc05069-4c24-40a7-976e-8b87ed915541\"},{\"content\":{\"connectorIds\":[],\"side\":\"HIDDEN\"},\"type\":\"ConnectorPlacement.EquallySpacedRectSide\",\"uuid\":\"da030f82-010e-483f-97d7-c36c3edfce40\"}]},\"type\":\"ConnectorPlacement.EquallySpacedConnector\",\"uuid\":\"1bb0f634-fa5d-4f47-8259-a0e02a201bbc\"}],\"packageUris\":[\"http://schema.mathworks.com/mf0/Connector/R2020b\"],\"version\":\"1.0\"}"
  Voltage Measurement : spsVoltageMeasurementLib/Voltage Measurement  PhasorSimulation=off  OutputType=Complex  PSBequivalent=0
  p_gen : Constant  Value=400e3
  + : PMIOPort  Side=Right
  - : PMIOPort  Port=2  Side=Right
  m : Outport
  wires:
  Switch/1 -> Controlled Current Source/1
  Constant4/1 -> Switch/3
  Divide/1 -> Switch/1
  VI measurement/1 -> m/1
  Voltage Measurement/1 -> Divide/2
  p_gen/1 -> Divide/1
  Clock/1 -> 1-D Lookup Table1/1
  enable/1 -> AND/1
  AND/1 -> Switch/2
  1-D Lookup Table1/1 -> AND/2
  connections:
  VI measurement/LConn1 -- Voltage Measurement/LConn1 -- +/RConn1
  VI measurement/LConn2 -- Voltage Measurement/LConn2 -- -/RConn1
  VI measurement/RConn2 -- Controlled Current Source/LConn1
  Controlled Current Source/RConn1 -- VI measurement/RConn1

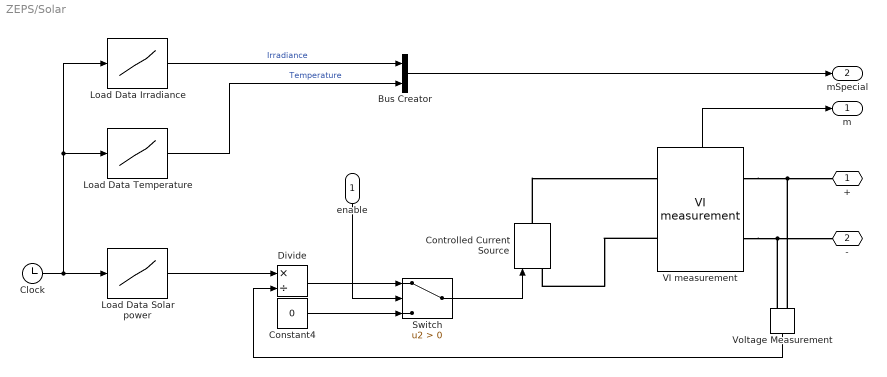
== system ZEPS/Solar ==
  enable : Inport
  Bus Creator : BusCreator  Inputs=2
  Clock : Clock
  Constant4 : Constant  Value=0
  Controlled Current Source : spsControlledCurrentSourceLib/Controlled Current Source  Initialize=on  Source_Type=AC  Amplitude=0  Phase=0  Frequency=0  Measurements=None
  Divide : Product  Inputs=*/
  Load Data Irradiance : Lookup_n-D  NumberOfTableDimensions=1  BreakpointsForDimension1=sun.time  BeginIndexSearchUsingPreviousIndexResult=on  Table=sun.irradiance  InternalRulePriority=Speed  RndMeth=Simplest  InputSameDT=on
  Load Data Solar power : Lookup_n-D  NumberOfTableDimensions=1  BreakpointsForDimension1=sun.time  BeginIndexSearchUsingPreviousIndexResult=on  Table=sun.power  InternalRulePriority=Speed  RndMeth=Simplest  InputSameDT=on
  Load Data Temperature : Lookup_n-D  NumberOfTableDimensions=1  BreakpointsForDimension1=sun.time  BeginIndexSearchUsingPreviousIndexResult=on  Table=sun.temperature  InternalRulePriority=Speed  RndMeth=Simplest  InputSameDT=on
  Switch : Switch  Criteria=u2 > Threshold
  VI measurement : mylib/VI measurement  SystemSampleTime=-1  VariantActivationTime=update diagram  Latency=0  AutoFrameSizeCalculation=off
      settings: PortSchema="{\"entries\":[{\"content\":{\"sides\":[{\"content\":{\"connectorIds\":[\"LConn1\",\"LConn2\"]},\"type\":\"ConnectorPlacement.EquallySpacedRectSide\",\"uuid\":\"f3b73344-d0cf-4b93-ad96-f780fa5a1256\"},{\"content\":{\"connectorIds\":[\"RConn1\",\"RConn2\"],\"side\":\"RIGHT\"},\"type\":\"ConnectorPlacement.EquallySpacedRectSide\",\"uuid\":\"030ebb8c-daa3-4185-a78c-b002204e2a62\"},{\"content\":{\"connectorIds\":[\"Out1\"],\"side\":\"TOP\"},\"type\":\"ConnectorPlacement.EquallySpacedRectSide\",\"uuid\":\"0cc05069-4c24-40a7-976e-8b87ed915541\"},{\"content\":{\"connectorIds\":[],\"side\":\"HIDDEN\"},\"type\":\"ConnectorPlacement.EquallySpacedRectSide\",\"uuid\":\"da030f82-010e-483f-97d7-c36c3edfce40\"}]},\"type\":\"ConnectorPlacement.EquallySpacedConnector\",\"uuid\":\"1bb0f634-fa5d-4f47-8259-a0e02a201bbc\"}],\"packageUris\":[\"http://schema.mathworks.com/mf0/Connector/R2020b\"],\"version\":\"1.0\"}"
  Voltage Measurement : spsVoltageMeasurementLib/Voltage Measurement  PhasorSimulation=off  OutputType=Complex  PSBequivalent=0
  + : PMIOPort  Side=Right
  - : PMIOPort  Port=2  Side=Right
  m : Outport
  mSpecial : Outport  Port=2
  wires:
  enable/1 -> Switch/2
  Divide/1 -> Switch/1
  Clock/1 -> Load Data Solar power/1, Load Data Temperature/1, Load Data Irradiance/1
  Switch/1 -> Controlled Current Source/1
  Constant4/1 -> Switch/3
  VI measurement/1 -> m/1
  Load Data Solar power/1 -> Divide/1
  Voltage Measurement/1 -> Divide/2
  Load Data Irradiance/1 -> Bus Creator/1  "Irradiance"
  Load Data Temperature/1 -> Bus Creator/2  "Temperature"
  Bus Creator/1 -> mSpecial/1
  connections:
  VI measurement/LConn1 -- Voltage Measurement/LConn1 -- +/RConn1
  VI measurement/LConn2 -- Voltage Measurement/LConn2 -- -/RConn1
  VI measurement/RConn2 -- Controlled Current Source/LConn1
  Controlled Current Source/RConn1 -- VI measurement/RConn1

== system ZEPS/Waste Water ==
  enable : Inport
  AC converter simple : mylib/AC converter simple  eff=0.98
  Constant : Constant  Value=0
  Power : Constant  Value=1000
  Switch : Switch  Criteria=u2 > Threshold
  VI measurement : mylib/VI measurement  SystemSampleTime=-1  VariantActivationTime=update diagram  Latency=0  AutoFrameSizeCalculation=off
      settings: PortSchema="{\"entries\":[{\"content\":{\"sides\":[{\"content\":{\"connectorIds\":[\"LConn1\",\"LConn2\"]},\"type\":\"ConnectorPlacement.EquallySpacedRectSide\",\"uuid\":\"f3b73344-d0cf-4b93-ad96-f780fa5a1256\"},{\"content\":{\"connectorIds\":[\"RConn1\",\"RConn2\"],\"side\":\"RIGHT\"},\"type\":\"ConnectorPlacement.EquallySpacedRectSide\",\"uuid\":\"030ebb8c-daa3-4185-a78c-b002204e2a62\"},{\"content\":{\"connectorIds\":[\"Out1\"],\"side\":\"TOP\"},\"type\":\"ConnectorPlacement.EquallySpacedRectSide\",\"uuid\":\"0cc05069-4c24-40a7-976e-8b87ed915541\"},{\"content\":{\"connectorIds\":[],\"side\":\"HIDDEN\"},\"type\":\"ConnectorPlacement.EquallySpacedRectSide\",\"uuid\":\"da030f82-010e-483f-97d7-c36c3edfce40\"}]},\"type\":\"ConnectorPlacement.EquallySpacedConnector\",\"uuid\":\"1bb0f634-fa5d-4f47-8259-a0e02a201bbc\"}],\"packageUris\":[\"http://schema.mathworks.com/mf0/Connector/R2020b\"],\"version\":\"1.0\"}"
  +Vdc : PMIOPort  Tag=PMCPort  Side=Left
  -Vdc : PMIOPort  Tag=PMCPort  Port=2  Side=Left
  m : Outport
  wires:
  VI measurement/1 -> m/1
  enable/1 -> Switch/2
  Constant/1 -> Switch/3
  Power/1 -> Switch/1
  Switch/1 -> AC converter simple/1
  connections:
  VI measurement/LConn1 -- AC converter simple/RConn1
  VI measurement/LConn2 -- AC converter simple/RConn2
  +Vdc/RConn1 -- VI measurement/RConn1
  -Vdc/RConn1 -- VI measurement/RConn2

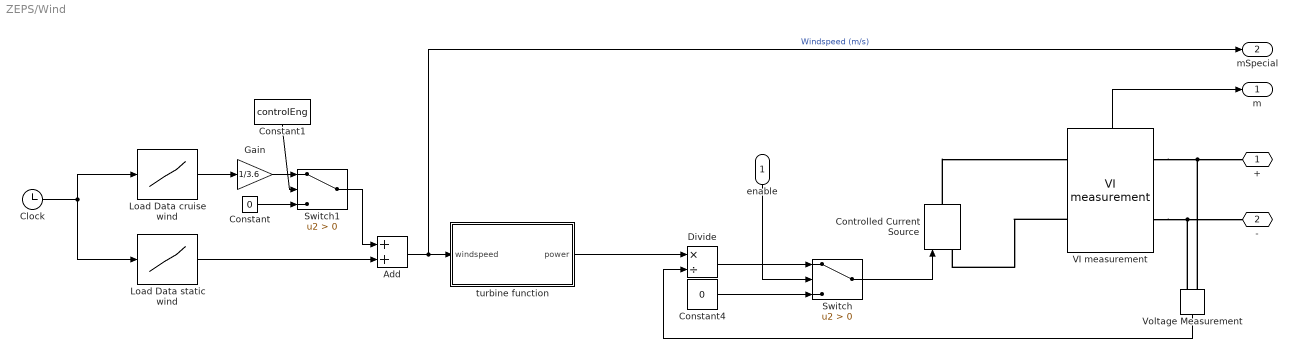
== system ZEPS/Wind ==
  enable : Inport
  Add : Sum
  Clock : Clock
  Constant : Constant  Value=0
  Constant1 : Constant  Value=controlEng
  Constant4 : Constant  Value=0
  Controlled Current Source : spsControlledCurrentSourceLib/Controlled Current Source  Initialize=on  Source_Type=AC  Amplitude=0  Phase=0  Frequency=0  Measurements=None
  Divide : Product  Inputs=*/
  Gain : Gain  Gain=1/3.6
  Load Data cruise wind : Lookup_n-D  NumberOfTableDimensions=1  BreakpointsForDimension1=data.time  BeginIndexSearchUsingPreviousIndexResult=on  Table=data.Speedkmh  InternalRulePriority=Speed  RndMeth=Simplest  InputSameDT=on
  Load Data static wind : Lookup_n-D  NumberOfTableDimensions=1  BreakpointsForDimension1=sun.time  BeginIndexSearchUsingPreviousIndexResult=on  Table=sun.windspeed  InternalRulePriority=Speed  RndMeth=Simplest  InputSameDT=on
  Switch : Switch  Criteria=u2 > Threshold
  Switch1 : Switch  Criteria=u2 > Threshold
  VI measurement : mylib/VI measurement  SystemSampleTime=-1  VariantActivationTime=update diagram  Latency=0  AutoFrameSizeCalculation=off
      settings: PortSchema="{\"entries\":[{\"content\":{\"sides\":[{\"content\":{\"connectorIds\":[\"LConn1\",\"LConn2\"]},\"type\":\"ConnectorPlacement.EquallySpacedRectSide\",\"uuid\":\"f3b73344-d0cf-4b93-ad96-f780fa5a1256\"},{\"content\":{\"connectorIds\":[\"RConn1\",\"RConn2\"],\"side\":\"RIGHT\"},\"type\":\"ConnectorPlacement.EquallySpacedRectSide\",\"uuid\":\"030ebb8c-daa3-4185-a78c-b002204e2a62\"},{\"content\":{\"connectorIds\":[\"Out1\"],\"side\":\"TOP\"},\"type\":\"ConnectorPlacement.EquallySpacedRectSide\",\"uuid\":\"0cc05069-4c24-40a7-976e-8b87ed915541\"},{\"content\":{\"connectorIds\":[],\"side\":\"HIDDEN\"},\"type\":\"ConnectorPlacement.EquallySpacedRectSide\",\"uuid\":\"da030f82-010e-483f-97d7-c36c3edfce40\"}]},\"type\":\"ConnectorPlacement.EquallySpacedConnector\",\"uuid\":\"1bb0f634-fa5d-4f47-8259-a0e02a201bbc\"}],\"packageUris\":[\"http://schema.mathworks.com/mf0/Connector/R2020b\"],\"version\":\"1.0\"}"
  Voltage Measurement : spsVoltageMeasurementLib/Voltage Measurement  PhasorSimulation=off  OutputType=Complex  PSBequivalent=0
  turbine function : Subsystem
  + : PMIOPort  Side=Right
  - : PMIOPort  Port=2  Side=Right
  m : Outport
  mSpecial : Outport  Port=2
  wires:
  Switch/1 -> Controlled Current Source/1
  enable/1 -> Switch/2
  Constant4/1 -> Switch/3
  Divide/1 -> Switch/1
  turbine function/1(power) -> Divide/1
  VI measurement/1 -> m/1
  Voltage Measurement/1 -> Divide/2
  Clock/1 -> Load Data cruise wind/1, Load Data static wind/1
  Load Data cruise wind/1 -> Gain/1
  Load Data static wind/1 -> Add/2
  Add/1 -> mSpecial/1, turbine function/1(windspeed)  "Windspeed (m/s)"
  Gain/1 -> Switch1/1
  Switch1/1 -> Add/1
  Constant/1 -> Switch1/3
  Constant1/1 -> Switch1/2
  connections:
  VI measurement/LConn1 -- Voltage Measurement/LConn1 -- +/RConn1
  VI measurement/LConn2 -- Voltage Measurement/LConn2 -- -/RConn1
  VI measurement/RConn2 -- Controlled Current Source/LConn1
  Controlled Current Source/RConn1 -- VI measurement/RConn1

== system ZEPS/untitledPanel1 ==
  Bow Thruster : ToggleSwitchBlock  Tag=HiddenForWebPanel  PanelInfo="{\"panelId\":\"panelId-675edb10-d60a-4e4f-998b-78dbe922e38f\",\"type\":\"panelChild\",\"version\":\"2019b\",\"zIndex\":1500006}"  LabelPosition=Bottom
      settings: Values={{'Off', 'On'}, [0 1]}
  Engines : ToggleSwitchBlock  Tag=HiddenForWebPanel  PanelInfo="{\"panelId\":\"panelId-675edb10-d60a-4e4f-998b-78dbe922e38f\",\"type\":\"panelChild\",\"version\":\"2019b\",\"zIndex\":1500012}"  LabelPosition=Bottom
      settings: Values={{'Off', 'On'}, [0 1]}
  Fresh Water : ToggleSwitchBlock  Tag=HiddenForWebPanel  PanelInfo="{\"panelId\":\"panelId-675edb10-d60a-4e4f-998b-78dbe922e38f\",\"type\":\"panelChild\",\"version\":\"2019b\",\"zIndex\":1500008}"  LabelPosition=Bottom
      settings: Values={{'Off', 'On'}, [0 1]}
  Fuel Cells : ToggleSwitchBlock  Tag=HiddenForWebPanel  PanelInfo="{\"panelId\":\"panelId-675edb10-d60a-4e4f-998b-78dbe922e38f\",\"type\":\"panelChild\",\"version\":\"2019b\",\"zIndex\":1500002}"
      settings: Values={{'Off', 'On'}, [0 1]}
  Hotel Services : ToggleSwitchBlock  Tag=HiddenForWebPanel  PanelInfo="{\"panelId\":\"panelId-675edb10-d60a-4e4f-998b-78dbe922e38f\",\"type\":\"panelChild\",\"version\":\"2019b\",\"zIndex\":1500004}"  LabelPosition=Bottom
      settings: Values={{'Off', 'On'}, [0 1]}
  Solar : ToggleSwitchBlock  Tag=HiddenForWebPanel  PanelInfo="{\"panelId\":\"panelId-675edb10-d60a-4e4f-998b-78dbe922e38f\",\"type\":\"panelChild\",\"version\":\"2019b\",\"zIndex\":1500014}"
      settings: Values={{'Off', 'On'}, [0 1]}
  Waste Water : ToggleSwitchBlock  Tag=HiddenForWebPanel  PanelInfo="{\"panelId\":\"panelId-675edb10-d60a-4e4f-998b-78dbe922e38f\",\"type\":\"panelChild\",\"version\":\"2019b\",\"zIndex\":1500010}"  LabelPosition=Bottom
      settings: Values={{'Off', 'On'}, [0 1]}
  Wind : ToggleSwitchBlock  Tag=HiddenForWebPanel  PanelInfo="{\"panelId\":\"panelId-675edb10-d60a-4e4f-998b-78dbe922e38f\",\"type\":\"panelChild\",\"version\":\"2019b\",\"zIndex\":1500016}"
      settings: Values={{'Off', 'On'}, [0 1]}
  panelInfo : PanelWebBlock  Tag=HiddenForWebPanel  PanelInfo="{\"compacted\":false,\"height\":214,\"isActiveTab\":true,\"labels\":{},\"left\":5,\"name\":\"untitledPanel1\",\"panelId\":\"panelId-675edb10-d60a-4e4f-998b-78dbe922e38f\",\"tabIndex\":0,\"tabbedSetId\":\"tabbedSet2494630049\",\"top\":5,\"type\":\"panel\",\"version\":\"2019b\",\"visible\":true,\"width\":304,\"zIndex\":1500004}"

== system ZEPS/Engines/propeller function ==
  RPM : Inport
  Activation : Inport  Port=2
  Constant : Constant  Value=0
  activation : Switch  Threshold=600
  limit : Saturate  UpperLimit=1200  LowerLimit=-inf
  n3 : Product  Inputs=***
  p : Constant  Value=0.00017222
  propeller : Product  Inputs=**  RndMeth=Zero  SaturateOnIntegerOverflow=on
  rpm : Outport
  P : Outport  Port=2
  wires:
  Constant/1 -> activation/3
  n3/1 -> propeller/2
  p/1 -> propeller/1
  RPM/1 -> limit/1
  activation/1 -> n3/3, n3/1, n3/2
  propeller/1 -> P/1
  limit/1 -> rpm/1, activation/1
  Activation/1 -> activation/2

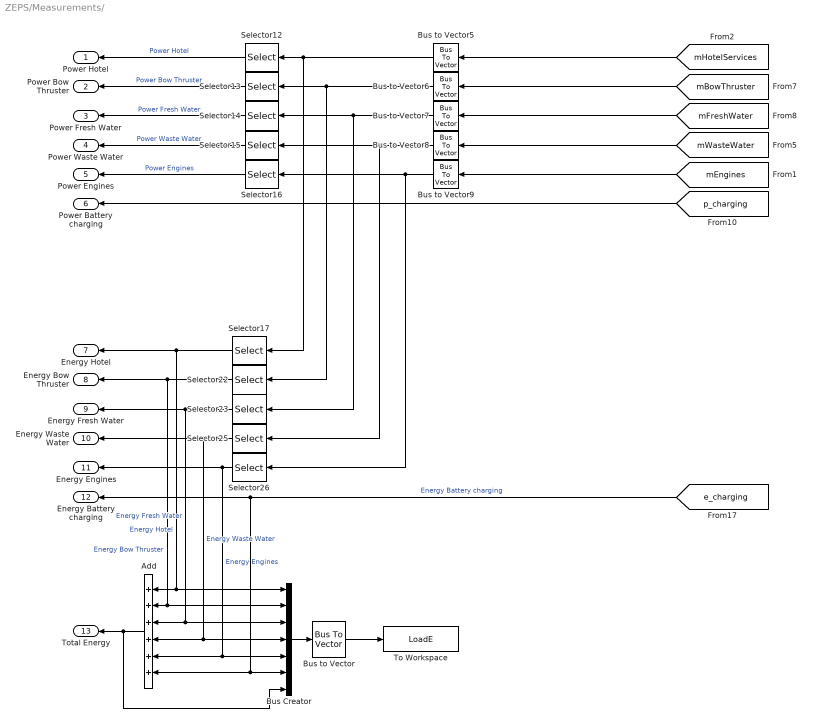
== system ZEPS/Measurements/  ==
  Add : Sum  Inputs=++++++
  Bus Creator : BusCreator  Inputs=7
  Bus to Vector{,5..9} (6 alike) : BusToVector
  Selector{12..16} (5 alike) : Selector  InputPortWidth=4  IndexOptions=Index vector (dialog)  Indices=[3]  OutputSizes=1
  Selector{17,22..23,25..26} (5 alike) : Selector  InputPortWidth=4  IndexOptions=Index vector (dialog)  Indices=4  OutputSizes=1
  To Workspace : ToWorkspace  VariableName=LoadE  SaveFormat=Timeseries  SampleTime=3600
  Power Hotel : Outport
  Power Bow Thruster : Outport  Port=2
  Power Fresh Water : Outport  Port=3
  Power Waste Water : Outport  Port=4
  Power Engines : Outport  Port=5
  Power Battery charging : Outport  Port=6
  Energy Hotel : Outport  Port=7
  Energy Bow Thruster : Outport  Port=8
  Energy Fresh Water : Outport  Port=9
  Energy Waste Water : Outport  Port=10
  Energy Engines : Outport  Port=11
  Energy Battery charging : Outport  Port=12
  Total Energy : Outport  Port=13
  wires:
  Selector16/1 -> Power Engines/1  "Power Engines"
  Selector15/1 -> Power Waste Water/1  "Power Waste Water"
  [mFreshWater] -> Bus to Vector7/1
  [mBowThruster] -> Bus to Vector6/1
  Selector12/1 -> Power Hotel/1  "Power Hotel"
  [mHotelServices] -> Bus to Vector5/1
  Selector17/1 -> Energy Hotel/1, Add/1, Bus Creator/1  "Energy Hotel"
  Bus to Vector5/1 -> Selector17/1, Selector12/1
  Add/1 -> Bus Creator/7, Total Energy/1
  Selector13/1 -> Power Bow Thruster/1  "Power Bow Thruster"
  Selector23/1 -> Energy Fresh Water/1, Add/3, Bus Creator/3  "Energy Fresh Water"
  Selector22/1 -> Energy Bow Thruster/1, Add/2, Bus Creator/2  "Energy Bow Thruster"
  Selector26/1 -> Energy Engines/1, Add/5, Bus Creator/5  "Energy Engines"
  [mEngines] -> Bus to Vector9/1
  [mWasteWater] -> Bus to Vector8/1
  Selector25/1 -> Energy Waste Water/1, Add/4, Bus Creator/4  "Energy Waste Water"
  Selector14/1 -> Power Fresh Water/1  "Power Fresh Water"
  [p_charging] -> Power Battery charging/1
  Bus to Vector6/1 -> Selector13/1, Selector22/1
  Bus to Vector7/1 -> Selector14/1, Selector23/1
  Bus to Vector8/1 -> Selector15/1, Selector25/1
  Bus to Vector9/1 -> Selector16/1, Selector26/1
  [e_charging] -> Energy Battery charging/1, Add/6, Bus Creator/6  "Energy Battery charging"
  Bus Creator/1 -> Bus to Vector/1
  Bus to Vector/1 -> To Workspace/1

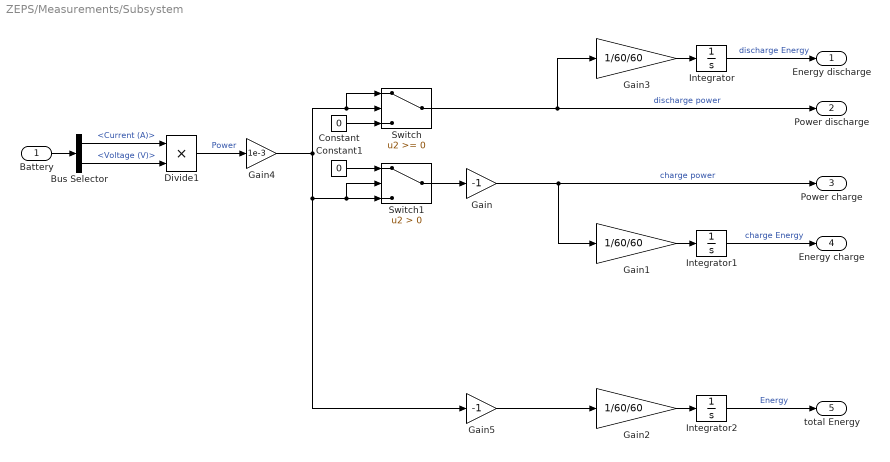
== system ZEPS/Measurements/Subsystem ==
  Battery : Inport
  Bus Selector : BusSelector  OutputSignals=Current (A),Voltage (V)
  Constant : Constant  Value=0
  Constant1 : Constant  Value=0
  Divide1 : Product  Inputs=**
  Gain : Gain  Gain=-1
  Gain1 : Gain  Gain=1/60/60
  Gain2 : Gain  Gain=1/60/60
  Gain3 : Gain  Gain=1/60/60
  Gain4 : Gain  Gain=1e-3
  Gain5 : Gain  Gain=-1
  Integrator : Integrator
  Integrator1 : Integrator
  Integrator2 : Integrator
  Switch : Switch
  Switch1 : Switch  Criteria=u2 > Threshold
  Energy discharge : Outport
  Power discharge : Outport  Port=2
  Power charge : Outport  Port=3
  Energy charge : Outport  Port=4
  total Energy : Outport  Port=5
  wires:
  Battery/1 -> Bus Selector/1
  Bus Selector/1 -> Divide1/1  "<Current (A)>"
  Bus Selector/2 -> Divide1/2  "<Voltage (V)>"
  Constant/1 -> Switch/3
  Constant1/1 -> Switch1/1
  Divide1/1 -> Gain4/1  "Power"
  Gain3/1 -> Integrator/1
  Switch/1 -> Gain3/1, Power discharge/1  "discharge power"
  Gain1/1 -> Integrator1/1
  Integrator/1 -> Energy discharge/1  "discharge Energy"
  Integrator1/1 -> Energy charge/1  "charge Energy"
  Switch1/1 -> Gain/1
  Gain/1 -> Gain1/1, Power charge/1  "charge power"
  Integrator2/1 -> total Energy/1  "Energy"
  Gain2/1 -> Integrator2/1
  Gain4/1 -> Gain5/1, Switch1/3, Switch1/2, Switch/1, Switch/2
  Gain5/1 -> Gain2/1

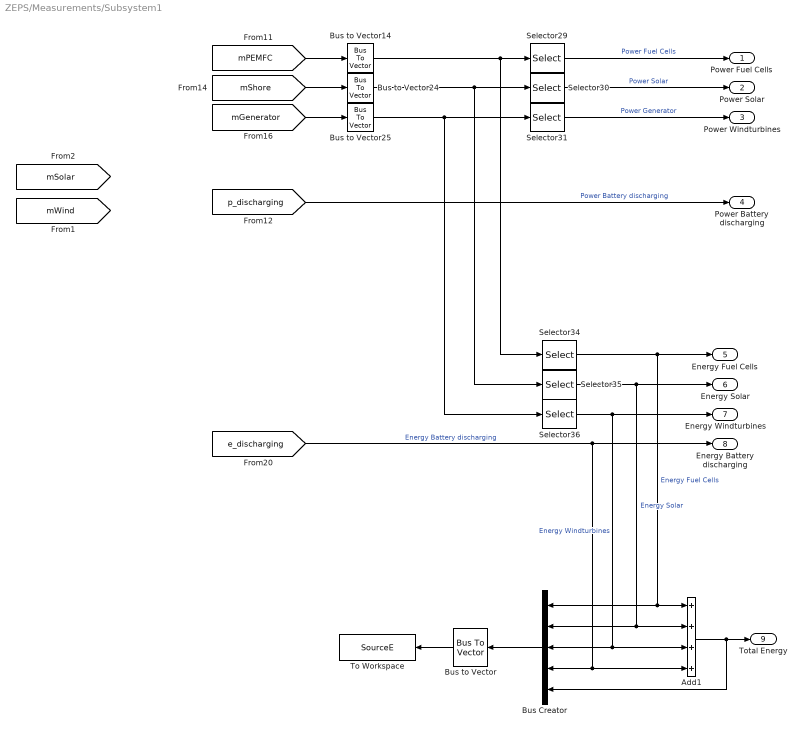
== system ZEPS/Measurements/Subsystem1 ==
  Add1 : Sum  Inputs=++++
  Bus Creator : BusCreator  Inputs=5
  Bus to Vector{,14,24..25} (4 alike) : BusToVector
  Selector29 : Selector  InputPortWidth=4  IndexOptions=Index vector (dialog)  Indices=[3]  OutputSizes=1
  Selector30 : Selector  InputPortWidth=4  IndexOptions=Index vector (dialog)  Indices=[3]  OutputSizes=1
  Selector31 : Selector  InputPortWidth=4  IndexOptions=Index vector (dialog)  Indices=[3]  OutputSizes=1
  Selector34 : Selector  InputPortWidth=4  IndexOptions=Index vector (dialog)  Indices=4  OutputSizes=1
  Selector35 : Selector  InputPortWidth=4  IndexOptions=Index vector (dialog)  Indices=4  OutputSizes=1
  Selector36 : Selector  InputPortWidth=4  IndexOptions=Index vector (dialog)  Indices=4  OutputSizes=1
  To Workspace : ToWorkspace  VariableName=SourceE  SaveFormat=Timeseries  SampleTime=3600
  Power Fuel Cells : Outport
  Power Solar : Outport  Port=2
  Power Windturbines : Outport  Port=3
  Power Battery discharging : Outport  Port=4
  Energy Fuel Cells : Outport  Port=5
  Energy Solar : Outport  Port=6
  Energy Windturbines : Outport  Port=7
  Energy Battery discharging : Outport  Port=8
  Total Energy : Outport  Port=9
  wires:
  Selector29/1 -> Power Fuel Cells/1  "Power Fuel Cells"
  [p_discharging] -> Power Battery discharging/1  "Power Battery discharging"
  Add1/1 -> Bus Creator/5, Total Energy/1
  Selector30/1 -> Power Solar/1  "Power Solar"
  [mPEMFC] -> Bus to Vector14/1
  Bus to Vector25/1 -> Selector31/1, Selector36/1
  [e_discharging] -> Energy Battery discharging/1, Add1/4, Bus Creator/4  "Energy Battery discharging"
  Selector31/1 -> Power Windturbines/1  "Power Generator"
  Selector35/1 -> Energy Solar/1, Add1/2, Bus Creator/2  "Energy Solar"
  [mShore] -> Bus to Vector24/1
  [mGenerator] -> Bus to Vector25/1
  Selector34/1 -> Energy Fuel Cells/1, Add1/1, Bus Creator/1  "Energy Fuel Cells"
  Selector36/1 -> Energy Windturbines/1, Add1/3, Bus Creator/3  "Energy Windturbines"
  Bus to Vector24/1 -> Selector30/1, Selector35/1
  Bus to Vector14/1 -> Selector34/1, Selector29/1
  Bus Creator/1 -> Bus to Vector/1
  Bus to Vector/1 -> To Workspace/1

== system ZEPS/Measurements/Time conversion ==
  Clock : Clock
  Gain1 : Gain  Gain=1/60/60
  Gain2 : Gain  Gain=1/60/60/24
  Days : Outport
  Hours : Outport  Port=2
  wires:
  Gain2/1 -> Days/1
  Gain1/1 -> Hours/1
  Clock/1 -> Gain1/1, Gain2/1

== system ZEPS/Wind/turbine function ==
  windspeed : Inport
  Add : Sum
  N : Gain
  Saturation : Saturate  UpperLimit=14  LowerLimit=2.7
  b : Constant  Value=-840
  m : Gain  Gain=560
  power : Outport
  wires:
  b/1 -> Add/1
  m/1 -> Add/2
  windspeed/1 -> Saturation/1
  Saturation/1 -> m/1
  Add/1 -> N/1
  N/1 -> power/1
